simulink model "Model1"  (R2018b)
settings: Solver=ode4  StartTime=0.0  StopTime=600  FixedStep=0.01  RelTol=1e-3
values from neighbouring files (symbols this model uses):
  Qini = [q0;q1;q2;q3]    [initialize.m]
  wini = [0.2*pi/180;0.2*pi/180;0.2*pi/180]    [initialize.m]
settings Model: Creator=15821  LastModifiedBy=MSI-NB

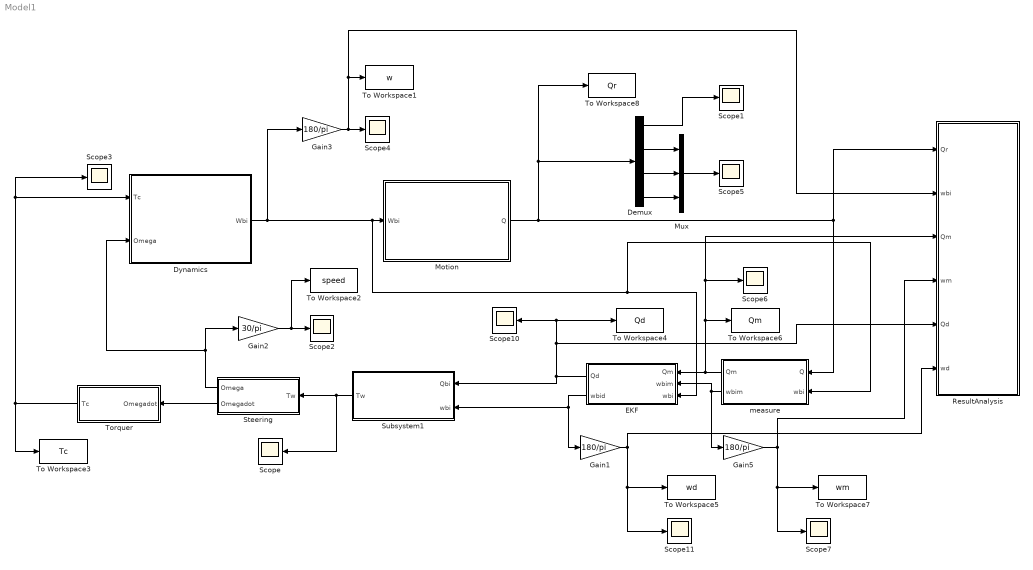
== system Model1 ==
  Demux : Demux
  Dynamics : Subsystem
  EKF : Subsystem
  Gain1 : Gain  Gain=180/pi
  Gain2 : Gain  Gain=30/pi
  Gain3 : Gain  Gain=180/pi
  Gain5 : Gain  Gain=180/pi
  Motion : Subsystem
  Mux : Mux  Inputs=3
  ResultAnalysis : Subsystem
  Scope{,1..7,10..11} (10 alike) : Scope
  Steering : Subsystem
  Subsystem1 : Subsystem
  To Workspace1 : ToWorkspace  VariableName=w  SaveFormat=Timeseries  SampleTime=-1
  To Workspace2 : ToWorkspace  VariableName=speed  SaveFormat=Timeseries  SampleTime=-1
  To Workspace3 : ToWorkspace  VariableName=Tc  SaveFormat=Timeseries  SampleTime=-1
  To Workspace4 : ToWorkspace  VariableName=Qd  SaveFormat=Timeseries  SampleTime=-1
  To Workspace5 : ToWorkspace  VariableName=wd  SaveFormat=Timeseries  SampleTime=-1
  To Workspace6 : ToWorkspace  VariableName=Qm  SaveFormat=Timeseries  SampleTime=-1
  To Workspace7 : ToWorkspace  VariableName=wm  SaveFormat=Timeseries  SampleTime=-1
  To Workspace8 : ToWorkspace  VariableName=Qr  SaveFormat=Timeseries  SampleTime=-1
  Torquer : Subsystem
  measure : Subsystem
  wires:
  Gain1/1 -> ResultAnalysis/6(wd), Scope11/1, To Workspace5/1
  Torquer/1(Tc) -> Dynamics/1(Tc), Scope3/1, To Workspace3/1
  measure/2(wbim) -> Gain5/1, EKF/2(wbim)
  Gain5/1 -> Scope7/1, To Workspace7/1, ResultAnalysis/4(wm)
  Dynamics/1(Wbi) -> Gain3/1, EKF/3(wbi), measure/2(wbi), Motion/1(Wbi)
  Demux/3 -> Mux/2
  EKF/2(wbid) -> Subsystem1/2(wbi), Gain1/1
  Motion/1(Q) -> ResultAnalysis/1(Qr), measure/1(Q), Demux/1, To Workspace8/1
  Demux/4 -> Mux/3
  Demux/1 -> Scope1/1
  measure/1(Qm) -> To Workspace6/1, ResultAnalysis/3(Qm), Scope6/1, EKF/1(Qm)
  Mux/1 -> Scope5/1
  Gain3/1 -> ResultAnalysis/2(wbi), To Workspace1/1, Scope4/1
  Demux/2 -> Mux/1
  Subsystem1/1(Tw) -> Scope/1, Steering/1(Tw)
  Steering/2(Omegadot) -> Torquer/1(Omegadot)
  Gain2/1 -> To Workspace2/1, Scope2/1
  EKF/1(Qd) -> Subsystem1/1(Qbi), Scope10/1, To Workspace4/1, ResultAnalysis/5(Qd)
  Steering/1(Omega) -> Gain2/1, Dynamics/2(Omega)

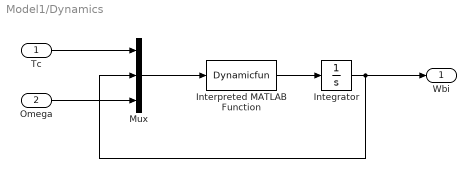
== system Model1/Dynamics ==
  Tc : Inport
  Omega : Inport  Port=2
  Integrator : Integrator  InitialCondition=wini
  Interpreted MATLAB Function : MATLABFcn  MATLABFcn=Dynamicfun  OutputDimensions=3
  Mux : Mux  Inputs=3
  Wbi : Outport
  wires:
  Mux/1 -> Interpreted MATLAB Function/1
  Tc/1 -> Mux/1
  Interpreted MATLAB Function/1 -> Integrator/1
  Integrator/1 -> Wbi/1, Mux/2
  Omega/1 -> Mux/3

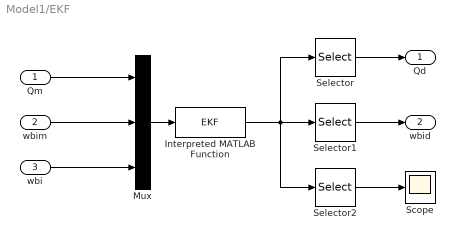
== system Model1/EKF ==
  Qm : Inport
  wbim : Inport  Port=2
  wbi : Inport  Port=3
  Interpreted MATLAB Function : MATLABFcn  MATLABFcn=EKF  OutputDimensions=8
  Mux : Mux  Inputs=3
  Scope : Scope
  Selector : Selector  InputPortWidth=8  IndexOptions=Index vector (dialog)  Indices=[1 2 3 4]  OutputSizes=1
  Selector1 : Selector  InputPortWidth=8  IndexOptions=Index vector (dialog)  Indices=[5 6 7]  OutputSizes=1
  Selector2 : Selector  InputPortWidth=8  IndexOptions=Index vector (dialog)  Indices=[8]  OutputSizes=1
  Qd : Outport
  wbid : Outport  Port=2
  wires:
  Mux/1 -> Interpreted MATLAB Function/1
  wbim/1 -> Mux/2
  Qm/1 -> Mux/1
  wbi/1 -> Mux/3
  Selector/1 -> Qd/1
  Interpreted MATLAB Function/1 -> Selector2/1, Selector1/1, Selector/1
  Selector1/1 -> wbid/1
  Selector2/1 -> Scope/1

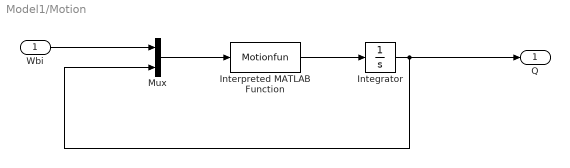
== system Model1/Motion ==
  Wbi : Inport
  Integrator : Integrator  InitialCondition=Qini
  Interpreted MATLAB Function : MATLABFcn  MATLABFcn=Motionfun  OutputDimensions=4
  Mux : Mux  Inputs=2
  Q : Outport
  wires:
  Interpreted MATLAB Function/1 -> Integrator/1
  Integrator/1 -> Q/1, Mux/2
  Mux/1 -> Interpreted MATLAB Function/1
  Wbi/1 -> Mux/1

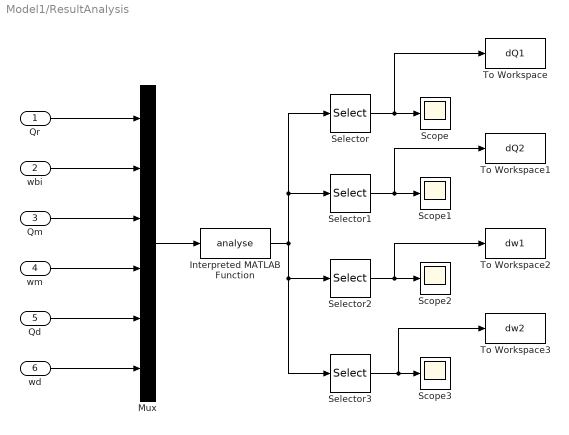
== system Model1/ResultAnalysis ==
  Qr : Inport
  wbi : Inport  Port=2
  Qm : Inport  Port=3
  wm : Inport  Port=4
  Qd : Inport  Port=5
  wd : Inport  Port=6
  Interpreted MATLAB Function : MATLABFcn  MATLABFcn=analyse  OutputDimensions=12
  Mux : Mux  Inputs=6
  Scope{,1..3} (4 alike) : Scope
  Selector : Selector  InputPortWidth=12  IndexOptions=Index vector (dialog)  Indices=[1 2 3]  OutputSizes=1
  Selector1 : Selector  InputPortWidth=12  IndexOptions=Index vector (dialog)  Indices=[4 5 6]  OutputSizes=1
  Selector2 : Selector  InputPortWidth=12  IndexOptions=Index vector (dialog)  Indices=[7 8 9]  OutputSizes=1
  Selector3 : Selector  InputPortWidth=12  IndexOptions=Index vector (dialog)  Indices=[10 11 12]  OutputSizes=1
  To Workspace : ToWorkspace  VariableName=dQ1  SaveFormat=Timeseries  SampleTime=-1
  To Workspace1 : ToWorkspace  VariableName=dQ2  SaveFormat=Timeseries  SampleTime=-1
  To Workspace2 : ToWorkspace  VariableName=dw1  SaveFormat=Timeseries  SampleTime=-1
  To Workspace3 : ToWorkspace  VariableName=dw2  SaveFormat=Timeseries  SampleTime=-1
  wires:
  Qr/1 -> Mux/1
  wbi/1 -> Mux/2
  Qm/1 -> Mux/3
  wm/1 -> Mux/4
  Qd/1 -> Mux/5
  wd/1 -> Mux/6
  Mux/1 -> Interpreted MATLAB Function/1
  Interpreted MATLAB Function/1 -> Selector3/1, Selector2/1, Selector1/1, Selector/1
  Selector/1 -> To Workspace/1, Scope/1
  Selector1/1 -> To Workspace1/1, Scope1/1
  Selector2/1 -> To Workspace2/1, Scope2/1
  Selector3/1 -> To Workspace3/1, Scope3/1

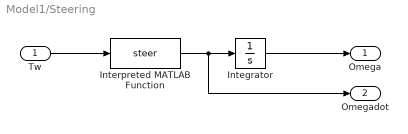
== system Model1/Steering ==
  Tw : Inport
  Integrator : Integrator
  Interpreted MATLAB Function : MATLABFcn  MATLABFcn=steer  OutputDimensions=4
  Omega : Outport
  Omegadot : Outport  Port=2
  wires:
  Tw/1 -> Interpreted MATLAB Function/1
  Interpreted MATLAB Function/1 -> Omegadot/1, Integrator/1
  Integrator/1 -> Omega/1

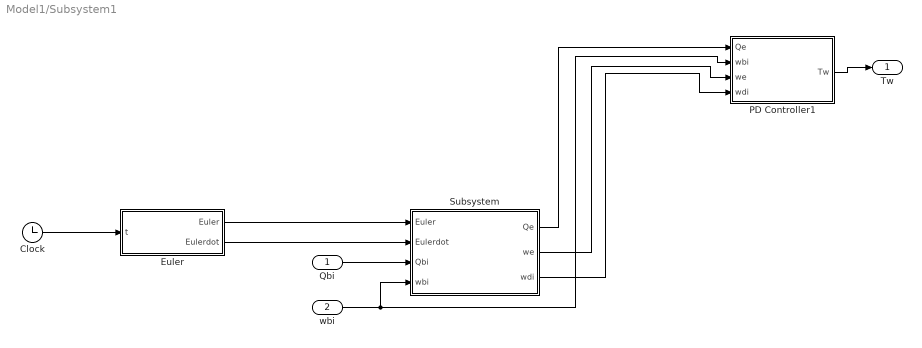
== system Model1/Subsystem1 ==
  Qbi : Inport
  wbi : Inport  Port=2
  Clock : Clock
  Euler : Subsystem
  PD Controller1 : Subsystem
  Subsystem : Subsystem
  Tw : Outport
  wires:
  Euler/2(Eulerdot) -> Subsystem/2(Eulerdot)
  Subsystem/2(we) -> PD Controller1/3(we)
  Euler/1(Euler) -> Subsystem/1(Euler)
  Subsystem/1(Qe) -> PD Controller1/1(Qe)
  Subsystem/3(wdi) -> PD Controller1/4(wdi)
  Clock/1 -> Euler/1(t)
  Qbi/1 -> Subsystem/3(Qbi)
  wbi/1 -> PD Controller1/2(wbi), Subsystem/4(wbi)
  PD Controller1/1(Tw) -> Tw/1

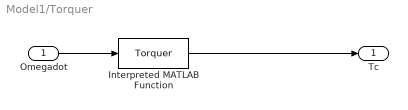
== system Model1/Torquer ==
  Omegadot : Inport
  Interpreted MATLAB Function : MATLABFcn  MATLABFcn=Torquer  OutputDimensions=3
  Tc : Outport
  wires:
  Omegadot/1 -> Interpreted MATLAB Function/1
  Interpreted MATLAB Function/1 -> Tc/1

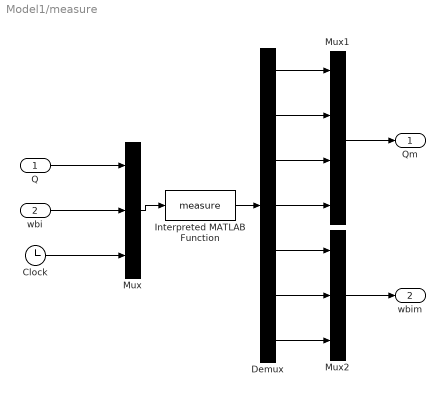
== system Model1/measure ==
  Q : Inport
  wbi : Inport  Port=2
  Clock : Clock
  Demux : Demux  Outputs=7
  Interpreted MATLAB Function : MATLABFcn  MATLABFcn=measure  OutputDimensions=7
  Mux : Mux  Inputs=3
  Mux1 : Mux
  Mux2 : Mux  Inputs=3
  Qm : Outport
  wbim : Outport  Port=2
  wires:
  Mux/1 -> Interpreted MATLAB Function/1
  Interpreted MATLAB Function/1 -> Demux/1
  Demux/4 -> Mux1/4
  Demux/3 -> Mux1/3
  Demux/2 -> Mux1/2
  Demux/1 -> Mux1/1
  Mux1/1 -> Qm/1
  Demux/5 -> Mux2/1
  Demux/6 -> Mux2/2
  Demux/7 -> Mux2/3
  Mux2/1 -> wbim/1
  wbi/1 -> Mux/2
  Q/1 -> Mux/1
  Clock/1 -> Mux/3

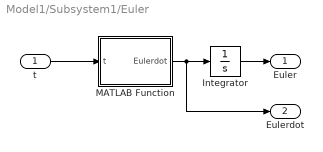
== system Model1/Subsystem1/Euler ==
  t : Inport
  Integrator : Integrator  InitialCondition=[-pi/8;pi/12;pi/6]
  MATLAB Function : MATLAB Function  TreatAsAtomicUnit=on
  Euler : Outport
  Eulerdot : Outport  Port=2
  wires:
  t/1 -> MATLAB Function/1(t)
  MATLAB Function/1(Eulerdot) -> Eulerdot/1, Integrator/1
  Integrator/1 -> Euler/1

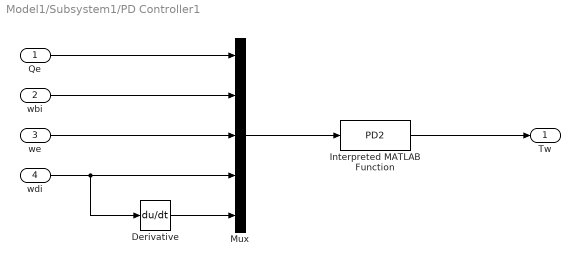
== system Model1/Subsystem1/PD Controller1 ==
  Qe : Inport
  wbi : Inport  Port=2
  we : Inport  Port=3
  wdi : Inport  Port=4
  Derivative : Derivative
  Interpreted MATLAB Function : MATLABFcn  MATLABFcn=PD2  OutputDimensions=3
  Mux : Mux  Inputs=5
  Tw : Outport
  wires:
  Mux/1 -> Interpreted MATLAB Function/1
  Interpreted MATLAB Function/1 -> Tw/1
  Qe/1 -> Mux/1
  wbi/1 -> Mux/2
  we/1 -> Mux/3
  wdi/1 -> Derivative/1, Mux/4
  Derivative/1 -> Mux/5

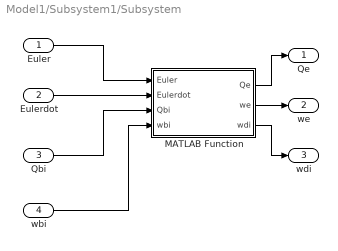
== system Model1/Subsystem1/Subsystem ==
  Euler : Inport
  Eulerdot : Inport  Port=2
  Qbi : Inport  Port=3
  wbi : Inport  Port=4
  MATLAB Function : MATLAB Function  TreatAsAtomicUnit=on
  Qe : Outport
  we : Outport  Port=2
  wdi : Outport  Port=3
  wires:
  Euler/1 -> MATLAB Function/1(Euler)
  Eulerdot/1 -> MATLAB Function/2(Eulerdot)
  Qbi/1 -> MATLAB Function/3(Qbi)
  wbi/1 -> MATLAB Function/4(wbi)
  MATLAB Function/2(we) -> we/1
  MATLAB Function/1(Qe) -> Qe/1
  MATLAB Function/3(wdi) -> wdi/1

== matlab function Model1/Subsystem1/Euler/MATLAB Function ==
  data: t input; Eulerdot output
function Eulerdot = fcn(t)

phidot = pi/4*0.08*pi*cos(0.08*pi*t-pi/6);
thetadot = pi/6*0.08*pi*cos(0.08*pi*t+pi/6);
psidot = -pi/6*0.08*pi*sin(0.08*pi*t);
Eulerdot = [phidot;thetadot;psidot];

== matlab function Model1/Subsystem1/Subsystem/MATLAB Function ==
  data: Euler input; Qe output; Eulerdot input; Qbi input; we output; wdi output; wbi input
function [Qe,we,wdi] = fcn(Euler,Eulerdot,Qbi,wbi)

Qdi = EulerToQ(Euler);
qdi0 = Qdi(1);
qdi = Qdi(2:4);
qbi0 = Qbi(1);
qbi = Qbi(2:4);
qe0 = qbi0*qdi0+qbi'*qdi;
qe = qdi0*qbi-qbi0*qdi+cross(qbi,qdi);
Qe = [qe0;qe];
EULER = [Euler;Eulerdot];
wdi = EulerdotToOmega(EULER);
Abd = (qe0^2-qe'*qe)*eye(3)+2*(qe*qe')-2*qe0*crossfun(qe);
we = wbi-Abd*wdi;
end
